simulink model "Single_Phase_Half_Wave_Controlled_with_battery_charger"  (R2020a)
settings: Solver=ode23tb  StartTime=0.0  StopTime=.06  MaxStep=3e-8  RelTol=1e-3
InitFcn:
  | a=0;
libraries: powerlib x7
settings Model: Creator=User  LastModifiedBy=User

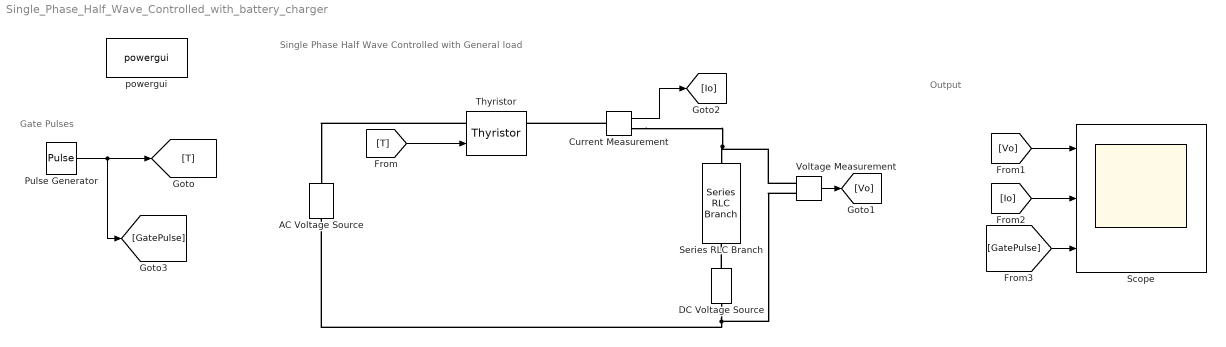
== system Single_Phase_Half_Wave_Controlled_with_battery_charger ==
  note: Gate Pulses
  note: Single Phase Half Wave Controlled with General load
  note: Output
  AC Voltage Source : powerlib/Electrical Sources/AC Voltage Source  Amplitude=100*sqrt(2)  Phase=0  Frequency=50  SampleTime=0  Measurements=None  BusType=swing  Pref=10e3  Qref=0  Qmin=-inf  Qmax=+inf
  Current Measurement : powerlib/Measurements/Current Measurement  PhasorSimulation=off  OutputType=Complex  PSBequivalent=0
  DC Voltage Source : powerlib/Electrical Sources/DC Voltage Source  Amplitude=40  Measurements=None
  Pulse Generator : DiscretePulseGenerator  PulseType=Time based  Period=.02  PulseWidth=5  PhaseDelay=(a/360)*.02
  Scope : Scope  NumInputPorts=3
  Series RLC Branch : powerlib/Elements/Series RLC Branch  LConnTagsString=__new0  RConnTagsString=__new0  BranchType=RL  Resistance=100  Inductance=100e-3  SetiL0=off  InitialCurrent=0  Capacitance=1e-6  Setx0=off  InitialVoltage=0  Measurements=None
  Thyristor : powerlib/Power Electronics/Thyristor  Ron=0.001  Lon=0  Vf=0.8  IC=0  Rs=500  Cs=250e-9  Measurements=on
  Voltage Measurement : powerlib/Measurements/Voltage Measurement  PhasorSimulation=off  OutputType=Complex  PSBequivalent=0
  powergui : powerlib/powergui  Priority=1  SimulationMode=Continuous  SampleTime=50e-6  frequency=60  Iterations=50  frequencyindice=50  Pbase=100e6  ErrMax=1e-4  UnitsV=kV  UnitsW=MW  buscounter=0  FunctionMessages=off  echomessages=off  EnableUseOfTLC=off  CurrentSourceSwitches=off  DisableSnubberDevices=on  DisableRonSwitches=on  DisableVfSwitches=on  DisplayEquations=off  AutomaticDiscreteSolvers=off  SolverType=Tustin/Backward Euler (TBE)  Interpol=off  ExternalGateDelay=off  methode=off  Ts=100  x0status=blocks  SPID=on  SwTol=0  HookPort=off  NonlinearTolerance=1e-4  nMaxIteration=100  ContinueOnMaxIteration=off  RestoreLinks=warning  ResistiveCurrentMeasurement=off  Frange=[0:2:500]  Ylog=off  Xlog=on  ShowGrid=off  save=off  variable=ZData  structure=0  ZoomFFT=off  StartTime=0.0  cycles=1  DisplayStyle=1  fundamental=60  FreqAxis=off  MaxFrequency=1000  frequencyindicesteady=1  RmsSteady=1  display=off
  wires:
  Pulse Generator/1 -> [GatePulse], [T]
  [T] -> Thyristor/1
  Current Measurement/1 -> [Io]
  Voltage Measurement/1 -> [Vo]
  [Vo] -> Scope/1
  [Io] -> Scope/2
  [GatePulse] -> Scope/3
  connections:
  Current Measurement/RConn1 -- Voltage Measurement/LConn1 -- Series RLC Branch/RConn1
  Thyristor/LConn1 -- AC Voltage Source/RConn1
  Current Measurement/LConn1 -- Thyristor/RConn1
  DC Voltage Source/RConn1 -- Series RLC Branch/LConn1
  DC Voltage Source/LConn1 -- Voltage Measurement/LConn2 -- AC Voltage Source/LConn1
